simulink model "CodeGen"  (R2020a)
settings: Solver=FixedStepDiscrete  StartTime=0.0  StopTime=10.0  FixedStep=1  RelTol=1e-3
libraries: simulink x1
settings Model: Creator=ashok  LastModifiedBy=ashok
settings RTWCC: GenCodeOnly=on  GenerateReport=on  LaunchReport=on

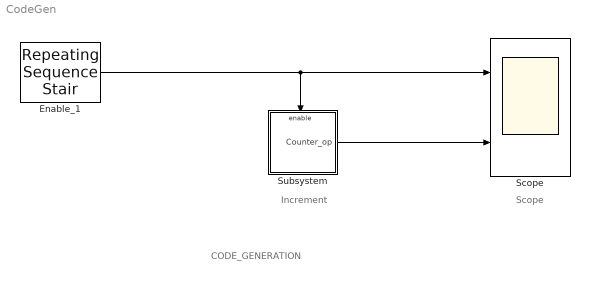
== system CodeGen ==
  note: CODE_GENERATION
  note: Scope
  note: Increment
  Enable_1 : simulink/Sources/Repeating Sequence Stair  OutValues=Enable_1  tsamp=-1  OutMin=[]  OutMax=[]  OutDataTypeStr=double  OutputDataTypeScalingMode=double  OutDataType=fixdt(0,8)  ConRadixGroup=Best Precision: Vector-wise  OutScaling=2^-12
  Scope : Scope  NumInputPorts=2
  Subsystem : Subsystem
  wires:
  Enable_1/1 -> Scope/1, Subsystem/Enable
  Subsystem/1(Counter_op) -> Scope/2

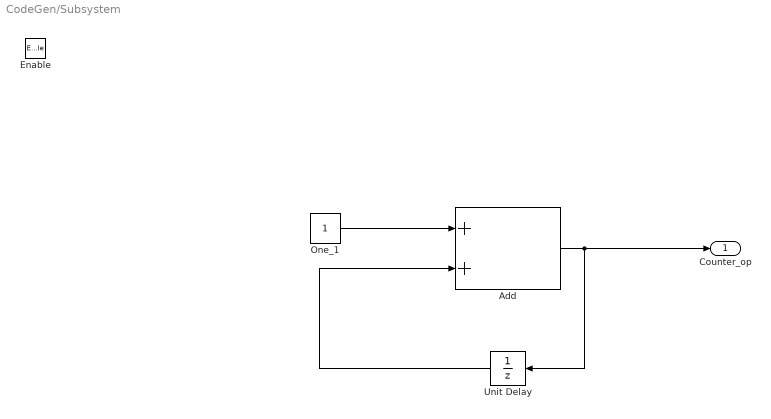
== system CodeGen/Subsystem ==
  Enable : EnablePort
  Add : Sum
  One_1 : Constant
  Unit Delay : UnitDelay  SampleTime=-1  HasFrameUpgradeWarning=on
  Counter_op : Outport
  wires:
  Add/1 -> Counter_op/1, Unit Delay/1
  Unit Delay/1 -> Add/2
  One_1/1 -> Add/1
